simulink model "MyPTControl_RTW"  (Simulink 10.3)
settings: Solver=ode1  StartTime=0.0  StopTime=inf  FixedStep=0.001  RelTol=1e-3
PreLoadFcn:
  | vehicle = 'Car'; if ~length(which('cmself')), cmenv; end
  | MyPTControl_RTW_bus
InitFcn:
  | vehicle = 'Car'; if ~length(which('cmself')), cmenv; end
  | MyPTControl_RTW_bus
undefined symbols (not defined in the file): EngineOut_Load, EngineOut_set_ISC, Ignition, ISGOut_Load, OperationState
libraries: simulink x11
(part 2 of 2)

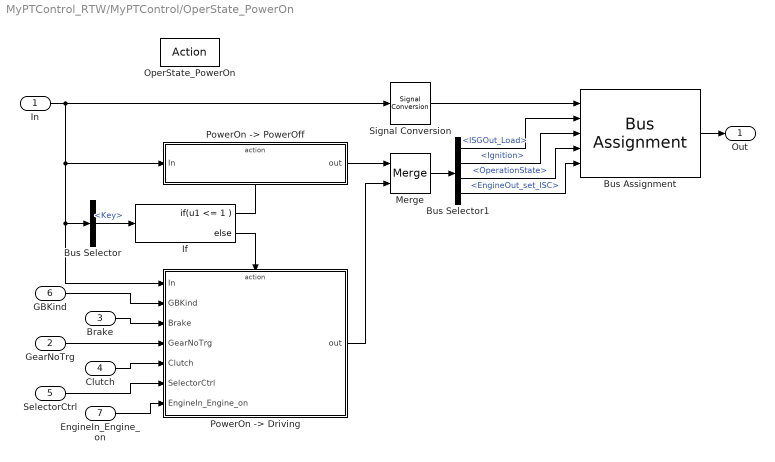
== system MyPTControl_RTW/MyPTControl/OperState_PowerOn ==
  In : Inport
  GearNoTrg : Inport  Port=2
  Brake : Inport  Port=3
  Clutch : Inport  Port=4
  SelectorCtrl : Inport  Port=5
  GBKind : Inport  Port=6
  EngineIn_Engine_on : Inport  Port=7
  OperState_PowerOn : ActionPort  ActionPortLabel=case [ 3 ]:
  Bus Assignment : BusAssignment  AssignedSignals=ISGOut_Load,Ignition,OperationState,EngineOut_set_ISC
  Bus Selector : BusSelector  OutputSignals=Key
  Bus Selector1 : BusSelector  OutputSignals=ISGOut_Load,Ignition,OperationState,EngineOut_set_ISC
  If : If  IfExpression=u1 <= 1
  Merge : Merge
  "PowerOn -> Driving" : Subsystem  TreatAsAtomicUnit=on
  "PowerOn -> PowerOff" : Subsystem  TreatAsAtomicUnit=on
  Signal Conversion : SignalConversion  ConversionOutput=Bus copy  OverrideOpt=off
  Out : Outport  VectorParamsAs1DForOutWhenUnconnected=off
  wires:
  Bus Selector1/4 -> Bus Assignment/5  "<EngineOut_set_ISC>"
  Signal Conversion/1 -> Bus Assignment/1
  "PowerOn -> PowerOff"/1(out) -> Merge/1
  SelectorCtrl/1 -> "PowerOn -> Driving"/6(SelectorCtrl)
  Clutch/1 -> "PowerOn -> Driving"/5(Clutch)
  EngineIn_Engine_on/1 -> "PowerOn -> Driving"/7(EngineIn_Engine_on)
  Bus Selector1/3 -> Bus Assignment/4  "<OperationState>"
  Bus Selector1/2 -> Bus Assignment/3  "<Ignition>"
  Bus Selector1/1 -> Bus Assignment/2  "<ISGOut_Load>"
  GearNoTrg/1 -> "PowerOn -> Driving"/4(GearNoTrg)
  Brake/1 -> "PowerOn -> Driving"/3(Brake)
  GBKind/1 -> "PowerOn -> Driving"/2(GBKind)
  Merge/1 -> Bus Selector1/1
  "PowerOn -> Driving"/1(out) -> Merge/2
  Bus Selector/1 -> If/1  "<Key>"
  Bus Assignment/1 -> Out/1
  In/1 -> Signal Conversion/1, "PowerOn -> PowerOff"/1(In), "PowerOn -> Driving"/1(In), Bus Selector/1
  If/2 -> "PowerOn -> Driving"/Action
  If/1 -> "PowerOn -> PowerOff"/Action

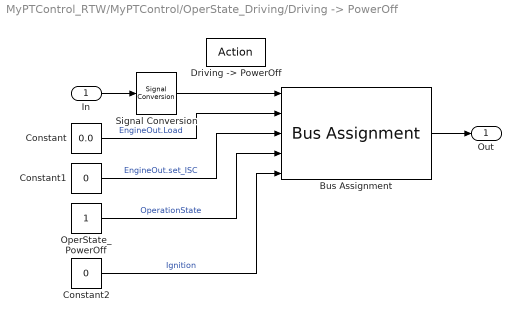
== system MyPTControl_RTW/MyPTControl/OperState_Driving/Driving -> PowerOff ==
  In : Inport
  "Driving -> PowerOff" : ActionPort  ActionPortLabel=elseif(u1<=1)
  Bus Assignment : BusAssignment  AssignedSignals=EngineOut_Load,EngineOut_set_ISC,Ignition,OperationState
  Constant : Constant  Value=0.0
  Constant1 : Constant  Value=0
  Constant2 : Constant  Value=0
  OperState_PowerOff : Constant
  Signal Conversion : SignalConversion  ConversionOutput=Bus copy  OverrideOpt=off
  Out : Outport  VectorParamsAs1DForOutWhenUnconnected=off
  wires:
  Signal Conversion/1 -> Bus Assignment/1
  Constant2/1 -> Bus Assignment/5  "Ignition"
  Constant/1 -> Bus Assignment/2  "EngineOut.Load"
  Bus Assignment/1 -> Out/1
  In/1 -> Signal Conversion/1
  OperState_PowerOff/1 -> Bus Assignment/4  "OperationState"
  Constant1/1 -> Bus Assignment/3  "EngineOut.set_ISC"

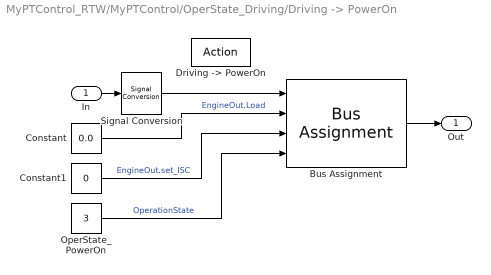
== system MyPTControl_RTW/MyPTControl/OperState_Driving/Driving -> PowerOn ==
  In : Inport
  "Driving -> PowerOn" : ActionPort  ActionPortLabel=if(~u2)
  Bus Assignment : BusAssignment  AssignedSignals=EngineOut_Load,EngineOut_set_ISC,OperationState
  Constant : Constant  Value=0.0
  Constant1 : Constant  Value=0
  OperState_PowerOn : Constant  Value=3
  Signal Conversion : SignalConversion  ConversionOutput=Bus copy  OverrideOpt=off
  Out : Outport  VectorParamsAs1DForOutWhenUnconnected=off
  wires:
  Signal Conversion/1 -> Bus Assignment/1
  Bus Assignment/1 -> Out/1
  In/1 -> Signal Conversion/1
  OperState_PowerOn/1 -> Bus Assignment/4  "OperationState"
  Constant1/1 -> Bus Assignment/3  "EngineOut.set_ISC"
  Constant/1 -> Bus Assignment/2  "EngineOut.Load"

== system MyPTControl_RTW/MyPTControl/OperState_Driving/If Action Subsystem1 ==
  In : Inport
  Gas : Inport  Port=2
  Action Port : ActionPort  ActionPortLabel=else
  Bus Assignment : BusAssignment  AssignedSignals=EngineOut_Load
  Gain1 : Gain
  Signal Conversion : SignalConversion  ConversionOutput=Bus copy  OverrideOpt=off
  Out : Outport  VectorParamsAs1DForOutWhenUnconnected=off
  wires:
  Signal Conversion/1 -> Bus Assignment/1
  Gain1/1 -> Bus Assignment/2  "EngineOut.Load"
  Bus Assignment/1 -> Out/1
  In/1 -> Signal Conversion/1
  Gas/1 -> Gain1/1

== system MyPTControl_RTW/MyPTControl/OperState_PowerOff/If Action Subsystem1 ==
  OperationState last cycle : Inport
  Action Port : ActionPort  ActionPortLabel=else
  OperationState : Outport  VectorParamsAs1DForOutWhenUnconnected=off
  wires:
  OperationState last cycle/1 -> OperationState/1

== system MyPTControl_RTW/MyPTControl/OperState_PowerOff/PowerOff -> Absent ==
  "PowerOff -> Absent" : ActionPort  ActionPortLabel=if(u1 == 0)
  OperState_Absent : Constant  Value=0
  OperationState : Outport  InitialOutput=0  VectorParamsAs1DForOutWhenUnconnected=off
  wires:
  OperState_Absent/1 -> OperationState/1

== system MyPTControl_RTW/MyPTControl/OperState_PowerOff/PowerOff -> PowerAcc ==
  "PowerOff -> PowerAcc" : ActionPort  ActionPortLabel=elseif(u1 >= 2)
  OperState_PowerAccesory : Constant  Value=2
  OperationState : Outport  InitialOutput=2  VectorParamsAs1DForOutWhenUnconnected=off
  wires:
  OperState_PowerAccesory/1 -> OperationState/1

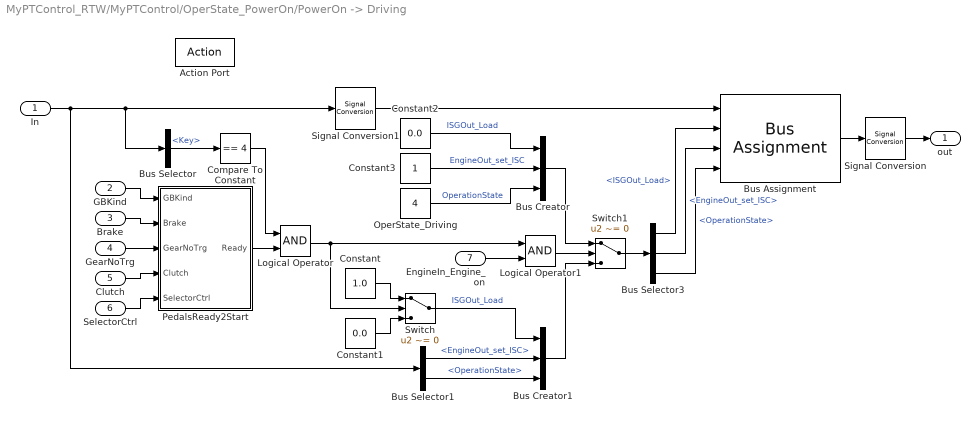
== system MyPTControl_RTW/MyPTControl/OperState_PowerOn/PowerOn -> Driving ==
  In : Inport
  GBKind : Inport  Port=2
  Brake : Inport  Port=3
  GearNoTrg : Inport  Port=4
  Clutch : Inport  Port=5
  SelectorCtrl : Inport  Port=6
  EngineIn_Engine_on : Inport  Port=7
  Action Port : ActionPort  ActionPortLabel=else
  Bus Assignment : BusAssignment  AssignedSignals=ISGOut_Load,EngineOut_set_ISC,OperationState
  Bus Creator : BusCreator  Inputs=3
  Bus Creator1 : BusCreator  Inputs=3
  Bus Selector : BusSelector  OutputSignals=Key
  Bus Selector1 : BusSelector  OutputSignals=EngineOut_set_ISC,OperationState
  Bus Selector3 : BusSelector  OutputSignals=ISGOut_Load,EngineOut_set_ISC,OperationState
  Compare To Constant : simulink/Logic and Bit Operations/Compare To Constant  relop===  const=4  OutDataTypeStr=uint8  ZeroCross=off
  Constant : Constant  Value=1.0
  Constant1 : Constant  Value=0.0
  Constant2 : Constant  Value=0.0
  Constant3 : Constant
  Logical Operator : Logic  AllPortsSameDT=off  OutDataTypeStr=boolean
  Logical Operator1 : Logic  AllPortsSameDT=off  OutDataTypeStr=boolean
  OperState_Driving : Constant  Value=4
  PedalsReady2Start : Subsystem
  Signal Conversion : SignalConversion  ConversionOutput=Bus copy  OverrideOpt=off
  Signal Conversion1 : SignalConversion  ConversionOutput=Bus copy  OverrideOpt=off
  Switch : Switch  Criteria=u2 ~= 0
  Switch1 : Switch  Criteria=u2 ~= 0
  out : Outport  VectorParamsAs1DForOutWhenUnconnected=off
  wires:
  Signal Conversion/1 -> out/1
  Bus Selector3/3 -> Bus Assignment/4  "<OperationState>"
  Bus Selector3/2 -> Bus Assignment/3  "<EngineOut_set_ISC>"
  Bus Selector3/1 -> Bus Assignment/2  "<ISGOut_Load>"
  Signal Conversion1/1 -> Bus Assignment/1
  Bus Assignment/1 -> Signal Conversion/1
  Constant3/1 -> Bus Creator/2  "EngineOut_set_ISC"
  Constant2/1 -> Bus Creator/1  "ISGOut_Load"
  OperState_Driving/1 -> Bus Creator/3  "OperationState"
  Bus Creator/1 -> Switch1/1
  Switch/1 -> Bus Creator1/1  "ISGOut_Load"
  Switch1/1 -> Bus Selector3/1
  Logical Operator1/1 -> Switch1/2
  Bus Creator1/1 -> Switch1/3
  Bus Selector1/2 -> Bus Creator1/3  "<OperationState>"
  Bus Selector1/1 -> Bus Creator1/2  "<EngineOut_set_ISC>"
  EngineIn_Engine_on/1 -> Logical Operator1/2
  Constant1/1 -> Switch/3
  Constant/1 -> Switch/1
  Logical Operator/1 -> Logical Operator1/1, Switch/2
  SelectorCtrl/1 -> PedalsReady2Start/5(SelectorCtrl)
  Clutch/1 -> PedalsReady2Start/4(Clutch)
  GearNoTrg/1 -> PedalsReady2Start/3(GearNoTrg)
  Brake/1 -> PedalsReady2Start/2(Brake)
  GBKind/1 -> PedalsReady2Start/1(GBKind)
  PedalsReady2Start/1(Ready) -> Logical Operator/2
  Compare To Constant/1 -> Logical Operator/1
  Bus Selector/1 -> Compare To Constant/1  "<Key>"
  In/1 -> Signal Conversion1/1, Bus Selector/1, Bus Selector1/1

== system MyPTControl_RTW/MyPTControl/OperState_PowerOn/PowerOn -> PowerOff ==
  In : Inport
  "PowerOn -> PowerOff" : ActionPort  ActionPortLabel=if(u1 <= 1 )
  Bus Assignment : BusAssignment  AssignedSignals=ISGOut_Load,Ignition,OperationState
  Constant : Constant  Value=0.0
  Constant1 : Constant  Value=0
  OperState_PowerOff : Constant
  Signal Conversion : SignalConversion  ConversionOutput=Bus copy  OverrideOpt=off
  out : Outport  VectorParamsAs1DForOutWhenUnconnected=off
  wires:
  Signal Conversion/1 -> Bus Assignment/1
  Bus Assignment/1 -> out/1
  In/1 -> Signal Conversion/1
  Constant1/1 -> Bus Assignment/3  "Ignition"
  Constant/1 -> Bus Assignment/2  "ISGOut_Load"
  OperState_PowerOff/1 -> Bus Assignment/4  "OperationState"

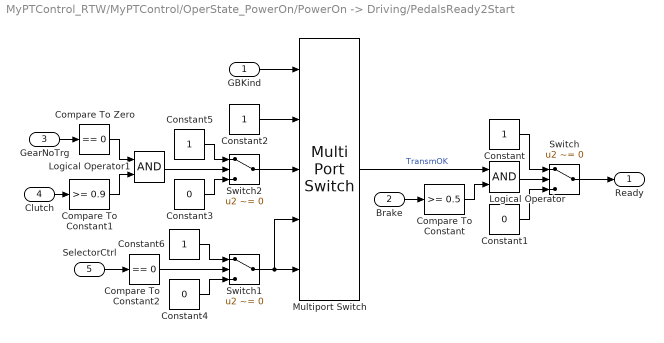
== system MyPTControl_RTW/MyPTControl/OperState_PowerOn/PowerOn -> Driving/PedalsReady2Start ==
  GBKind : Inport
  Brake : Inport  Port=2
  GearNoTrg : Inport  Port=3
  Clutch : Inport  Port=4
  SelectorCtrl : Inport  Port=5
  Compare To Constant : simulink/Logic and Bit Operations/Compare To Constant  relop=>=  const=0.5  OutDataTypeStr=uint8  ZeroCross=off
  Compare To Constant1 : simulink/Logic and Bit Operations/Compare To Constant  relop=>=  const=0.9  OutDataTypeStr=uint8  ZeroCross=off
  Compare To Constant2 : simulink/Logic and Bit Operations/Compare To Constant  relop===  const=0  OutDataTypeStr=uint8  ZeroCross=off
  Compare To Zero : simulink/Logic and Bit Operations/Compare To Zero  relop===  OutDataTypeStr=uint8  ZeroCross=off
  Constant{,2,5..6} (4 alike) : Constant
  Constant1 : Constant  Value=0
  Constant3 : Constant  Value=0
  Constant4 : Constant  Value=0
  Logical Operator : Logic  AllPortsSameDT=off  OutDataTypeStr=boolean
  Logical Operator1 : Logic  AllPortsSameDT=off  OutDataTypeStr=boolean
  Multiport Switch : MultiPortSwitch  DataPortOrder=Zero-based contiguous  Inputs=4  zeroidx=on
  Switch : Switch  Criteria=u2 ~= 0
  Switch1 : Switch  Criteria=u2 ~= 0
  Switch2 : Switch  Criteria=u2 ~= 0
  Ready : Outport  VectorParamsAs1DForOutWhenUnconnected=off
  wires:
  Compare To Constant2/1 -> Switch1/2
  SelectorCtrl/1 -> Compare To Constant2/1
  Compare To Constant1/1 -> Logical Operator1/2
  Compare To Zero/1 -> Logical Operator1/1
  GearNoTrg/1 -> Compare To Zero/1
  Clutch/1 -> Compare To Constant1/1
  Logical Operator1/1 -> Switch2/2
  Constant6/1 -> Switch1/1
  Constant5/1 -> Switch2/1
  Constant4/1 -> Switch1/3
  Constant3/1 -> Switch2/3
  Switch2/1 -> Multiport Switch/3
  Switch1/1 -> Multiport Switch/4, Multiport Switch/5
  Constant2/1 -> Multiport Switch/2
  Constant/1 -> Switch/1
  Constant1/1 -> Switch/3
  Logical Operator/1 -> Switch/2
  Switch/1 -> Ready/1
  Compare To Constant/1 -> Logical Operator/2
  Brake/1 -> Compare To Constant/1
  Multiport Switch/1 -> Logical Operator/1  "TransmOK"
  GBKind/1 -> Multiport Switch/1
